simulink model "SimulatorLQGmodel"  (R2024b)
settings: Solver=VariableStepAuto  StartTime=0.0  StopTime=10.0  RelTol=1e-3
values from neighbouring files (symbols this model uses):
  deadzone_parameters = [deadzone_lower,deadzone_higher, use_deadzone_compensation]    [SimulatorLQR.m]
  input_noise_power = 1    [CalculateBestInputs.m]    (also in SimulatorLQG.m = 10; SimulatorLQR.m = 10)
  K = lqr(A, B, Qr, Rr)    [CalculateBestInputs.m]    (also in IP_MACRO.m; LAB2_Analyze_system.m; SimulatorLQG.m; SimulatorLQR.m)
  L = lqe(A, G, C, Qe, Re)    [CalculateBestInputs.m]    (also in IP_MACRO.m; SimulatorLQG.m)
  output_noise_power = 100    [CalculateBestInputs.m]    (also in SimulatorLQG.m = 10; SimulatorLQR.m = 10)
  use_input_noise = 0    [CalculateBestInputs.m]    (also in SimulatorLQG.m = 1; SimulatorLQR.m)
  use_output_noise = 10    [CalculateBestInputs.m]    (also in SimulatorLQG.m = 1; SimulatorLQR.m = 0)
  x0 = [pi/2 0 0.1 0 0].'    [CalculateBestInputs.m]    (also in SimulatorLQG.m; SimulatorLQR.m = [1.3 0 -0.3 0 0].')
undefined symbols (not defined in the file or in its folder): A, B, C, D
libraries: simulink x2
settings Model: Creator=ricar  LastModifiedBy=ricar

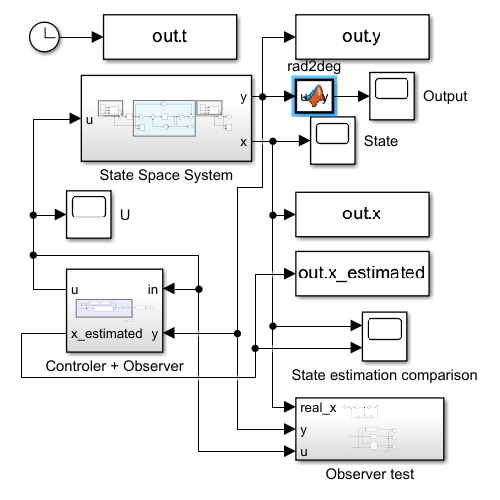
[thumbnail: Simulink's stored preview of the top-level diagram]
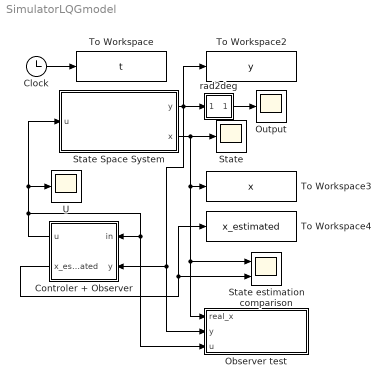
== system SimulatorLQGmodel ==
  Clock : Clock
  Controler + Observer : Subsystem
  Observer test : Subsystem
  Output : Scope
  State : Scope
  State Space System : Subsystem
  State estimation comparison : Scope  NumInputPorts=2
  To Workspace : ToWorkspace  VariableName=t  SampleTime=-1
  To Workspace2 : ToWorkspace  VariableName=y  SampleTime=-1
  To Workspace3 : ToWorkspace  VariableName=x  SampleTime=-1
  To Workspace4 : ToWorkspace  VariableName=x_estimated  SampleTime=-1
  U : Scope
  rad2deg : MATLAB Function  TreatAsAtomicUnit=on
  wires:
  Controler + Observer/1(u) -> State Space System/1(u), U/1, Observer test/3(u), Controler + Observer/1(in)
  State Space System/1(y) -> rad2deg/1(u), To Workspace2/1, Observer test/2(y), Controler + Observer/2(y)
  State Space System/2(x) -> State/1, To Workspace3/1, Observer test/1(real_x), State estimation comparison/1
  Clock/1 -> To Workspace/1
  Controler + Observer/2(x_estimated) -> To Workspace4/1, State estimation comparison/2
  rad2deg/1(y) -> Output/1

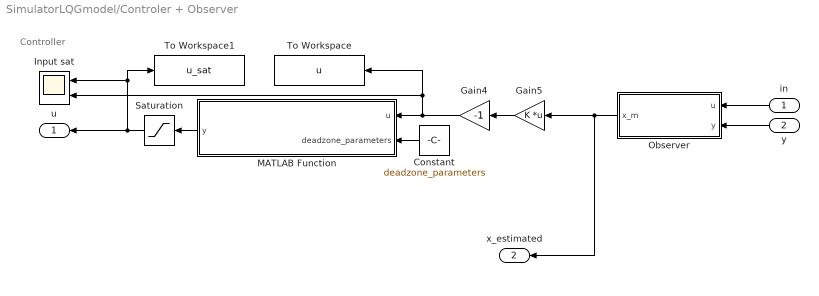
== system SimulatorLQGmodel/Controler + Observer ==
  note: Controller
  in : Inport
  y : Inport  Port=2
  Constant : Constant  Value=deadzone_parameters
  Gain4 : Gain  Gain=-1
  Gain5 : Gain  Gain=K  Multiplication=Matrix(K*u)
  Input sat : Scope  NumInputPorts=2
  MATLAB Function : MATLAB Function  TreatAsAtomicUnit=on
  Observer : Subsystem
  Saturation : Saturate  UpperLimit=5  LowerLimit=-5
  To Workspace : ToWorkspace  VariableName=u  SampleTime=-1
  To Workspace1 : ToWorkspace  VariableName=u_sat  SampleTime=-1
  u : Outport
  x_estimated : Outport  Port=2
  wires:
  MATLAB Function/1(y) -> Saturation/1
  Constant/1 -> MATLAB Function/2(deadzone_parameters)
  Saturation/1 -> u/1, Input sat/1, To Workspace1/1
  Gain4/1 -> To Workspace/1, Input sat/2, MATLAB Function/1(u)
  Gain5/1 -> Gain4/1
  Observer/1(x_m) -> x_estimated/1, Gain5/1
  in/1 -> Observer/1(u)
  y/1 -> Observer/2(y)

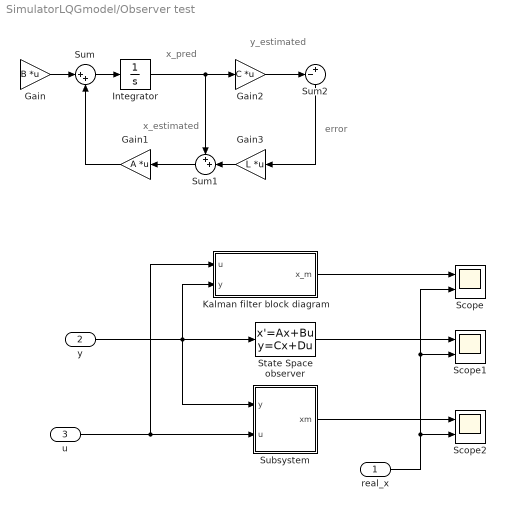
== system SimulatorLQGmodel/Observer test ==
  note: x_pred
  note: x_estimated
  note: y_estimated
  note: error
  real_x : Inport
  y : Inport  Port=2
  u : Inport  Port=3
  Gain : Gain  Gain=B  Multiplication=Matrix(K*u)
  Gain1 : Gain  Gain=A  Multiplication=Matrix(K*u)
  Gain2 : Gain  Gain=C  Multiplication=Matrix(K*u)
  Gain3 : Gain  Gain=L  Multiplication=Matrix(K*u)
  Integrator : Integrator  InitialCondition=x0
  Kalman filter block diagram : Subsystem
  Scope : Scope  NumInputPorts=2
  Scope1 : Scope  NumInputPorts=2
  Scope2 : Scope  NumInputPorts=2
  State Space observer : StateSpace  A=A - B * K - L * C  B=L  C=eye(5)  D=zeros(5,2)  InitialCondition=x0
  Subsystem : Subsystem
  Sum : Sum  Inputs=|++
  Sum1 : Sum  Inputs=++|
  Sum2 : Sum  Inputs=-+|
  wires:
  Integrator/1 -> Sum1/1, Gain2/1
  Gain1/1 -> Sum/2
  Gain/1 -> Sum/1
  Sum/1 -> Integrator/1
  Sum1/1 -> Gain1/1
  Gain3/1 -> Sum1/2
  Gain2/1 -> Sum2/1
  Sum2/1 -> Gain3/1
  u/1 -> Kalman filter block diagram/1(u), Subsystem/2(u)
  y/1 -> Subsystem/1(y), Kalman filter block diagram/2(y), State Space observer/1
  Kalman filter block diagram/1(x_m) -> Scope/1
  State Space observer/1 -> Scope1/1
  Subsystem/1(xm) -> Scope2/1
  real_x/1 -> Scope/2, Scope1/2, Scope2/2

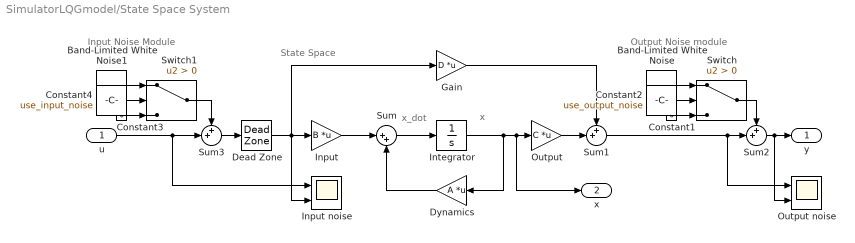
== system SimulatorLQGmodel/State Space System ==
  note: State Space
  note: Output Noise module
  note: Input Noise Module
  note: x_dot
  note: x
  u : Inport
  Band-Limited White Noise : simulink/Sources/Band-Limited White Noise  Cov=[0.000001*output_noise_power 0.000001*output_noise_power]  Ts=0.005  seed=[23341 2]
  Band-Limited White Noise1 : simulink/Sources/Band-Limited White Noise  Cov=[0.00001*input_noise_power]  Ts=0.01  seed=[145]
  Constant1 : Constant  Value=0
  Constant2 : Constant  Value=use_output_noise
  Constant3 : Constant  Value=0
  Constant4 : Constant  Value=use_input_noise
  Dead Zone : DeadZone  LowerValue=deadzone_lower  UpperValue=deadzone_higher  ZeroCross=off
  Dynamics : Gain  Gain=A  Multiplication=Matrix(K*u)
  Gain : Gain  Gain=D  Multiplication=Matrix(K*u)
  Input : Gain  Gain=B  Multiplication=Matrix(K*u)
  Input noise : Scope  NumInputPorts=2
  Integrator : Integrator  InitialCondition=x0
  Output : Gain  Gain=C  Multiplication=Matrix(K*u)
  Output noise : Scope  NumInputPorts=2
  Sum : Sum  Inputs=|++
  Sum1 : Sum  Inputs=++|
  Sum2 : Sum  Inputs=++|
  Sum3 : Sum  Inputs=++|
  Switch : Switch  Criteria=u2 > Threshold  SaturateOnIntegerOverflow=off  InputSameDT=off
  Switch1 : Switch  Criteria=u2 > Threshold  SaturateOnIntegerOverflow=off  InputSameDT=off
  y : Outport
  x : Outport  Port=2
  wires:
  Sum/1 -> Integrator/1
  Integrator/1 -> Dynamics/1, x/1, Output/1
  Input/1 -> Sum/1
  Dynamics/1 -> Sum/2
  Output/1 -> Sum1/2
  Gain/1 -> Sum1/1
  Sum1/1 -> Output noise/1, Sum2/2
  Sum2/1 -> y/1, Output noise/2
  Switch/1 -> Sum2/1
  Constant2/1 -> Switch/2
  Band-Limited White Noise/1 -> Switch/1
  Constant1/1 -> Switch/3
  Constant4/1 -> Switch1/2
  Switch1/1 -> Sum3/1
  Constant3/1 -> Switch1/3
  Band-Limited White Noise1/1 -> Switch1/1
  u/1 -> Input noise/1, Sum3/2
  Sum3/1 -> Dead Zone/1
  Dead Zone/1 -> Input noise/2, Gain/1, Input/1

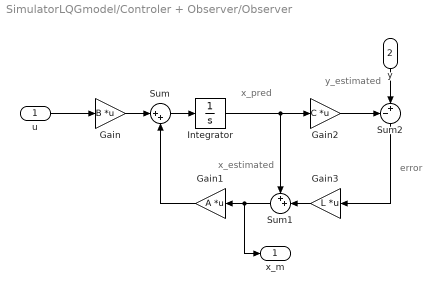
== system SimulatorLQGmodel/Controler + Observer/Observer ==
  note: x_estimated
  note: y_estimated
  note: x_pred
  note: error
  u : Inport
  y : Inport  Port=2
  Gain : Gain  Gain=B  Multiplication=Matrix(K*u)
  Gain1 : Gain  Gain=A  Multiplication=Matrix(K*u)
  Gain2 : Gain  Gain=C  Multiplication=Matrix(K*u)
  Gain3 : Gain  Gain=L  Multiplication=Matrix(K*u)
  Integrator : Integrator  InitialCondition=x0
  Sum : Sum  Inputs=|++
  Sum1 : Sum  Inputs=++|
  Sum2 : Sum  Inputs=-+|
  x_m : Outport
  wires:
  Gain2/1 -> Sum2/1
  Sum1/1 -> x_m/1, Gain1/1
  Sum2/1 -> Gain3/1
  Gain3/1 -> Sum1/2
  Gain/1 -> Sum/1
  Integrator/1 -> Sum1/1, Gain2/1
  Sum/1 -> Integrator/1
  Gain1/1 -> Sum/2
  u/1 -> Gain/1
  y/1 -> Sum2/2

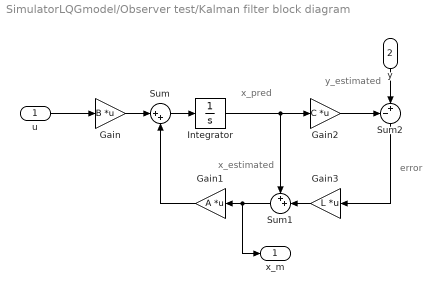
== system SimulatorLQGmodel/Observer test/Kalman filter block diagram ==
  note: x_estimated
  note: y_estimated
  note: x_pred
  note: error
  u : Inport
  y : Inport  Port=2
  Gain : Gain  Gain=B  Multiplication=Matrix(K*u)
  Gain1 : Gain  Gain=A  Multiplication=Matrix(K*u)
  Gain2 : Gain  Gain=C  Multiplication=Matrix(K*u)
  Gain3 : Gain  Gain=L  Multiplication=Matrix(K*u)
  Integrator : Integrator  InitialCondition=x0
  Sum : Sum  Inputs=|++
  Sum1 : Sum  Inputs=++|
  Sum2 : Sum  Inputs=-+|
  x_m : Outport
  wires:
  Gain2/1 -> Sum2/1
  Sum1/1 -> x_m/1, Gain1/1
  Sum2/1 -> Gain3/1
  Gain3/1 -> Sum1/2
  Gain/1 -> Sum/1
  Integrator/1 -> Sum1/1, Gain2/1
  Sum/1 -> Integrator/1
  Gain1/1 -> Sum/2
  u/1 -> Gain/1
  y/1 -> Sum2/2

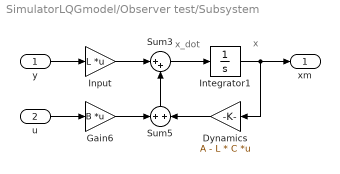
== system SimulatorLQGmodel/Observer test/Subsystem ==
  note: x_dot
  note: x
  y : Inport
  u : Inport  Port=2
  Dynamics : Gain  Gain=A - L * C  Multiplication=Matrix(K*u)
  Gain6 : Gain  Gain=B  Multiplication=Matrix(K*u)
  Input : Gain  Gain=L  Multiplication=Matrix(K*u)
  Integrator1 : Integrator  InitialCondition=x0
  Sum3 : Sum  Inputs=|++
  Sum5 : Sum  Inputs=+|+
  xm : Outport
  wires:
  Sum5/1 -> Sum3/2
  Dynamics/1 -> Sum5/2
  Sum3/1 -> Integrator1/1
  Input/1 -> Sum3/1
  Integrator1/1 -> Dynamics/1, xm/1
  Gain6/1 -> Sum5/1
  u/1 -> Gain6/1
  y/1 -> Input/1

== matlab function SimulatorLQGmodel/Controler + Observer/MATLAB Function ==
  data: u input; y output; deadzone_parameters input
function y = fcn(u,deadzone_parameters)
deadzone_low = deadzone_parameters(1);
deadzone_high = deadzone_parameters(2);
use_deadzone_compensation = deadzone_parameters(3);

deadzone_low = -0.38;
deadzone_high = 0.25;

if use_deadzone_compensation
    if u < deadzone_high && u > 0
        u = deadzone_high;

    elseif u > deadzone_low && u < 0
        u = deadzone_low;

    end
end
y = u;

== matlab function SimulatorLQGmodel/rad2deg ==
  data: u input; y output
function y = fcn(u)

y = rad2deg(u);
